simulink model "ImuCalibrator3Pass"  (R2018a)
settings: Solver=FixedStepDiscrete  StartTime=0.0  StopTime=inf  FixedStep=1/Fss  RelTol=1e-3
PreLoadFcn:
  | busDef
  | Fss = 1125;
  | Fss = 2100;
InitFcn:
  | modelDef = getModelDef(true);
undefined symbols (not defined in the file or in its folder): df, dw, Ggyr, Macc, Mgyr, numStates
libraries: simulink x15, vrlib x15, dspsigops x6, dspindex x6, dspinverses x6, dspstat3 x3, simulink_extras x3, dspmtrx3 x3, dspsrcs4 x3, dspmathops x3, dspswit3 x1
(part 3 of 4)

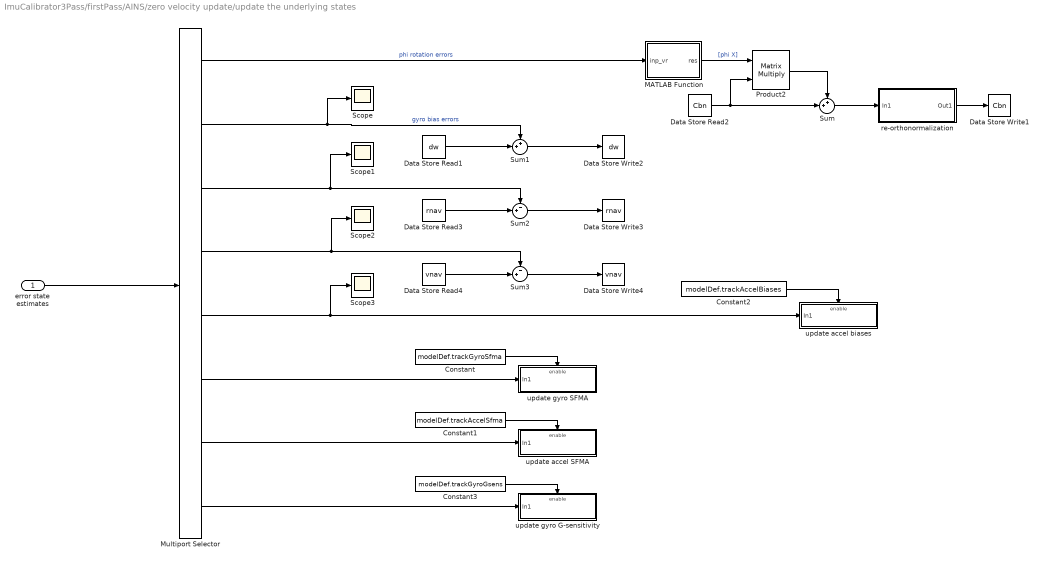
== system ImuCalibrator3Pass/firstPass/AINS/zero velocity update/update the underlying states ==
  " error state estimates" : Inport
  Constant : Constant  Value=modelDef.trackGyroSfma
  Constant1 : Constant  Value=modelDef.trackAccelSfma
  Constant2 : Constant  Value=modelDef.trackAccelBiases
  Constant3 : Constant  Value=modelDef.trackGyroGsens
  Data Store Read1 : DataStoreRead  DataStoreName=dw
  Data Store Read2 : DataStoreRead  DataStoreName=Cbn
  Data Store Read3 : DataStoreRead  DataStoreName=rnav
  Data Store Read4 : DataStoreRead  DataStoreName=vnav
  Data Store Write1 : DataStoreWrite  DataStoreName=Cbn
  Data Store Write2 : DataStoreWrite  DataStoreName=dw
  Data Store Write3 : DataStoreWrite  DataStoreName=rnav
  Data Store Write4 : DataStoreWrite  DataStoreName=vnav
  MATLAB Function : MATLAB Function  TreatAsAtomicUnit=on
  Multiport Selector : dspindex/Multiport Selector  rowsOrCols=Rows  idxCellArray={ 1:3, 4:6, 7:9, 10:12, 13:15, 16:24, 25:33, 34:42 }  idxErrMode=Clip Index
  Product2 : Product  Multiplication=Matrix(*)
  Scope{,1..3} (4 alike) : Scope
  Sum : Sum  Inputs=++|
  Sum1 : Sum  Inputs=++|
  Sum2 : Sum  Inputs=-+|
  Sum3 : Sum  Inputs=-+|
  re-orthonormalization : Subsystem  TreatAsAtomicUnit=on
  update accel SFMA : Subsystem
  update accel biases : Subsystem
  update gyro G-sensitivity : Subsystem
  update gyro SFMA : Subsystem
  wires:
  Multiport Selector/4 -> Sum3/1, Scope2/1
  Multiport Selector/3 -> Sum2/1, Scope1/1
  Sum3/1 -> Data Store Write4/1
  Data Store Read4/1 -> Sum3/2
  Data Store Read3/1 -> Sum2/2
  Sum2/1 -> Data Store Write3/1
  " error state estimates"/1 -> Multiport Selector/1
  Multiport Selector/2 -> Sum1/1, Scope/1  "gyro bias errors"
  Sum1/1 -> Data Store Write2/1
  Data Store Read1/1 -> Sum1/2
  Multiport Selector/1 -> MATLAB Function/1(inp_vr)  "phi rotation errors"
  re-orthonormalization/1(Out1) -> Data Store Write1/1
  Data Store Read2/1 -> Sum/2, Product2/2
  Sum/1 -> re-orthonormalization/1(In1)
  Product2/1 -> Sum/1
  MATLAB Function/1(res) -> Product2/1  "[phi X]"
  Constant/1 -> update gyro SFMA/Enable
  Multiport Selector/6 -> update gyro SFMA/1(In1)
  Constant1/1 -> update accel SFMA/Enable
  Multiport Selector/7 -> update accel SFMA/1(In1)
  Multiport Selector/5 -> update accel biases/1(In1), Scope3/1
  Constant2/1 -> update accel biases/Enable
  Constant3/1 -> update gyro G-sensitivity/Enable
  Multiport Selector/8 -> update gyro G-sensitivity/1(In1)

== system ImuCalibrator3Pass/secondPass/AINS/compass meas update/update the Cbn with the errors ==
  phi  rotation errors : Inport
  Data Store Read2 : DataStoreRead  DataStoreName=Cbn
  Data Store Write1 : DataStoreWrite  DataStoreName=Cbn
  MATLAB Function : MATLAB Function  TreatAsAtomicUnit=on
  Product2 : Product  Multiplication=Matrix(*)
  Sum : Sum  Inputs=++|
  re-orthonormalization : Subsystem  TreatAsAtomicUnit=on
  wires:
  MATLAB Function/1(res) -> Product2/1  "[phi X]"
  Product2/1 -> Sum/1
  Sum/1 -> re-orthonormalization/1(In1)
  phi  rotation errors/1 -> MATLAB Function/1(inp_vr)
  Data Store Read2/1 -> Product2/2, Sum/2
  re-orthonormalization/1(Out1) -> Data Store Write1/1

== system ImuCalibrator3Pass/secondPass/AINS/gravity meas update/update the Cbn and b_g with the errors ==
  " error state estimates" : Inport
  Data Store Read1 : DataStoreRead  DataStoreName=dw
  Data Store Read2 : DataStoreRead  DataStoreName=Cbn
  Data Store Read3 : DataStoreRead  DataStoreName=rnav
  Data Store Read4 : DataStoreRead  DataStoreName=vnav
  Data Store Read5 : DataStoreRead  DataStoreName=df
  Data Store Read6 : DataStoreRead  DataStoreName=Macc
  Data Store Read7 : DataStoreRead  DataStoreName=Mgyr
  Data Store Write1 : DataStoreWrite  DataStoreName=Cbn
  Data Store Write2 : DataStoreWrite  DataStoreName=dw
  Data Store Write3 : DataStoreWrite  DataStoreName=rnav
  Data Store Write4 : DataStoreWrite  DataStoreName=vnav
  Data Store Write5 : DataStoreWrite  DataStoreName=df
  Data Store Write6 : DataStoreWrite  DataStoreName=Macc
  Data Store Write7 : DataStoreWrite  DataStoreName=Mgyr
  MATLAB Function : MATLAB Function  TreatAsAtomicUnit=on
  Multiport Selector : dspindex/Multiport Selector  rowsOrCols=Rows  idxCellArray={ 1:3, 4:6, 7:9, 10:12, 13:15, 16:24, 25:33 }  idxErrMode=Clip Index
  Product2 : Product  Multiplication=Matrix(*)
  Reshape : Reshape  OutputDimensionality=Customize  OutputDimensions=[3,3]
  Reshape1 : Reshape  OutputDimensionality=Customize  OutputDimensions=[3,3]
  Sum{,1..6} (7 alike) : Sum  Inputs=++|
  re-orthonormalization : Subsystem  TreatAsAtomicUnit=on
  wires:
  Reshape1/1 -> Sum6/1
  Multiport Selector/7 -> Reshape1/1
  Reshape/1 -> Sum5/1
  Multiport Selector/6 -> Reshape/1
  Data Store Read7/1 -> Sum6/2
  Sum6/1 -> Data Store Write7/1
  Sum5/1 -> Data Store Write6/1
  Data Store Read6/1 -> Sum5/2
  Multiport Selector/5 -> Sum4/1
  Data Store Read5/1 -> Sum4/2
  Sum4/1 -> Data Store Write5/1
  Multiport Selector/4 -> Sum3/1
  Multiport Selector/3 -> Sum2/1
  Sum3/1 -> Data Store Write4/1
  Data Store Read4/1 -> Sum3/2
  Data Store Read3/1 -> Sum2/2
  Sum2/1 -> Data Store Write3/1
  " error state estimates"/1 -> Multiport Selector/1
  Multiport Selector/2 -> Sum1/1  "gyro bias errors"
  Sum1/1 -> Data Store Write2/1
  Data Store Read1/1 -> Sum1/2
  Multiport Selector/1 -> MATLAB Function/1(inp_vr)  "phi rotation errors"
  re-orthonormalization/1(Out1) -> Data Store Write1/1
  Data Store Read2/1 -> Sum/2, Product2/2
  Sum/1 -> re-orthonormalization/1(In1)
  Product2/1 -> Sum/1
  MATLAB Function/1(res) -> Product2/1  "[phi X]"

== system ImuCalibrator3Pass/secondPass/AINS/initialize states and covariances/INITIALIZED = 1 ==
  Enable : EnablePort  ShowOutputPort=on
  Constant : Constant
  Data Store Write : DataStoreWrite  DataStoreName=INITIALIZED
  Out1 : Outport  OutputWhenDisabled=reset  InitialOutput=false
  wires:
  Enable/1 -> Out1/1
  Constant/1 -> Data Store Write/1

== system ImuCalibrator3Pass/secondPass/AINS/initialize states and covariances/calc Cbn ==
  f^b : Inport
  Enable : EnablePort  ShowOutputPort=on
  Constant : Constant  Value=[1 0 0]
  Cross Product : vrlib/Utilities/Cross Product
      settings: SourceProductBaseCode=VR
  Cross Product1 : vrlib/Utilities/Cross Product
      settings: SourceProductBaseCode=VR
  Gain : Gain  Gain=-1
  Matrix Concatenate : Concatenate  NumInputs=3  Mode=Multidimensional array
  Normalize Vector : vrlib/Utilities/Normalize Vector  maxzero=0
      settings: SourceProductName=Simulink 3D Animation  SourceProductBaseCode=VR
  Normalize Vector1 : vrlib/Utilities/Normalize Vector  maxzero=0
      settings: SourceProductName=Simulink 3D Animation  SourceProductBaseCode=VR
  Normalize Vector2 : vrlib/Utilities/Normalize Vector  maxzero=0
      settings: SourceProductName=Simulink 3D Animation  SourceProductBaseCode=VR
  Out1 : Outport  OutputWhenDisabled=reset  InitialOutput=false
  Cbn : Outport  Port=2
  wires:
  Enable/1 -> Out1/1
  Matrix Concatenate/1 -> Cbn/1
  Normalize Vector2/1 -> Matrix Concatenate/3
  Normalize Vector1/1 -> Matrix Concatenate/2
  Normalize Vector/1 -> Matrix Concatenate/1
  Cross Product1/1 -> Normalize Vector/1  "north^b"
  Cross Product/1 -> Cross Product1/1, Normalize Vector1/1  "east^b"
  Constant/1 -> Cross Product/2
  Gain/1 -> Cross Product/1, Cross Product1/2, Normalize Vector2/1  "down^b"
  f^b/1 -> Gain/1  "up"

== system ImuCalibrator3Pass/secondPass/AINS/initialize states and covariances/set P ==
  Enable : EnablePort  ShowOutputPort=on
  Data Store Write : DataStoreWrite  DataStoreName=P
  Gain : Gain
  Gain2 : Gain
  Gain3 : Gain
  MATLAB Function1 : MATLAB Function  TreatAsAtomicUnit=on
  "initial position error, m rms" : Constant  Value=[0.01; 0.01; 0.01]  VectorParams1D=off
  "initial rotation error, rad rms" : Constant  Value=[0.1; 0.1; 0.1]  VectorParams1D=off
  "initial vel error, m/s" : Constant  Value=[0.01; 0.01; 0.01]  VectorParams1D=off
  Out1 : Outport  OutputWhenDisabled=reset  InitialOutput=false
  wires:
  Enable/1 -> Out1/1
  Gain3/1 -> MATLAB Function1/3(initialVelUncert)
  "initial vel error, m/s"/1 -> Gain3/1
  Gain2/1 -> MATLAB Function1/2(initialPosUncert)
  Gain/1 -> MATLAB Function1/1(initialRotUncert)
  "initial position error, m rms"/1 -> Gain2/1
  "initial rotation error, rad rms"/1 -> Gain/1
  MATLAB Function1/1(P0) -> Data Store Write/1

== system ImuCalibrator3Pass/secondPass/AINS/initialize states and covariances/set states ==
  Cbn : Inport
  Enable : EnablePort  ShowOutputPort=on
  Constant{,1..3} (4 alike) : Constant  Value=[0;0;0]
  Constant4 : Constant  Value=[0 0 0; 0 0 0; 0 0 0]  VectorParams1D=off
  Constant5 : Constant  Value=[0 0 0; 0 0 0; 0 0 0]  VectorParams1D=off
  Constant6 : Constant  Value=[1 0 0; 0 1 0; 0 0 1]  VectorParams1D=off
  Constant7 : Constant  Value=[1 0 0; 0 1 0; 0 0 1]  VectorParams1D=off
  Constant8 : Constant  Value=[0 0 0; 0 0 0; 0 0 0]  VectorParams1D=off
  Data Store Write : DataStoreWrite  DataStoreName=dw
  Data Store Write1 : DataStoreWrite  DataStoreName=df
  Data Store Write2 : DataStoreWrite  DataStoreName=vnav
  Data Store Write3 : DataStoreWrite  DataStoreName=rnav
  Data Store Write4 : DataStoreWrite  DataStoreName=Macc
  Data Store Write5 : DataStoreWrite  DataStoreName=Mgyr
  Data Store Write6 : DataStoreWrite  DataStoreName=IplusMinv_acc
  Data Store Write7 : DataStoreWrite  DataStoreName=IplusMinv_gyr
  Data Store Write8 : DataStoreWrite  DataStoreName=Cbn
  Data Store Write9 : DataStoreWrite  DataStoreName=Ggyr
  Out1 : Outport  OutputWhenDisabled=reset  InitialOutput=false
  wires:
  Constant8/1 -> Data Store Write9/1
  Cbn/1 -> Data Store Write8/1
  Enable/1 -> Out1/1
  Constant7/1 -> Data Store Write7/1
  Constant6/1 -> Data Store Write6/1
  Constant5/1 -> Data Store Write5/1
  Constant4/1 -> Data Store Write4/1
  Constant3/1 -> Data Store Write3/1
  Constant2/1 -> Data Store Write2/1
  Constant1/1 -> Data Store Write1/1
  Constant/1 -> Data Store Write/1

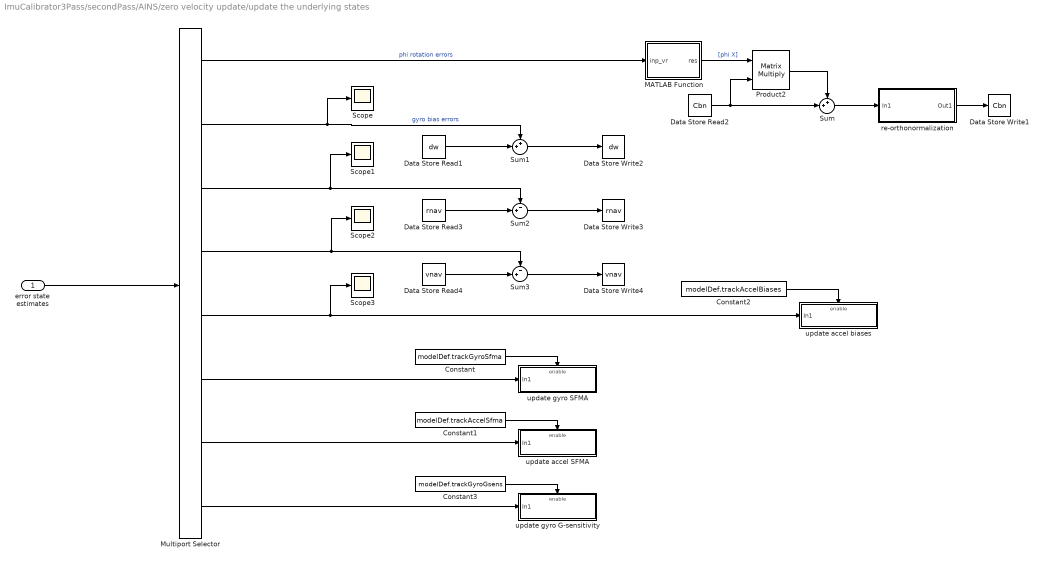
== system ImuCalibrator3Pass/secondPass/AINS/zero velocity update/update the underlying states ==
  " error state estimates" : Inport
  Constant : Constant  Value=modelDef.trackGyroSfma
  Constant1 : Constant  Value=modelDef.trackAccelSfma
  Constant2 : Constant  Value=modelDef.trackAccelBiases
  Constant3 : Constant  Value=modelDef.trackGyroGsens
  Data Store Read1 : DataStoreRead  DataStoreName=dw
  Data Store Read2 : DataStoreRead  DataStoreName=Cbn
  Data Store Read3 : DataStoreRead  DataStoreName=rnav
  Data Store Read4 : DataStoreRead  DataStoreName=vnav
  Data Store Write1 : DataStoreWrite  DataStoreName=Cbn
  Data Store Write2 : DataStoreWrite  DataStoreName=dw
  Data Store Write3 : DataStoreWrite  DataStoreName=rnav
  Data Store Write4 : DataStoreWrite  DataStoreName=vnav
  MATLAB Function : MATLAB Function  TreatAsAtomicUnit=on
  Multiport Selector : dspindex/Multiport Selector  rowsOrCols=Rows  idxCellArray={ 1:3, 4:6, 7:9, 10:12, 13:15, 16:24, 25:33, 34:42 }  idxErrMode=Clip Index
  Product2 : Product  Multiplication=Matrix(*)
  Scope{,1..3} (4 alike) : Scope
  Sum : Sum  Inputs=++|
  Sum1 : Sum  Inputs=++|
  Sum2 : Sum  Inputs=-+|
  Sum3 : Sum  Inputs=-+|
  re-orthonormalization : Subsystem  TreatAsAtomicUnit=on
  update accel SFMA : Subsystem
  update accel biases : Subsystem
  update gyro G-sensitivity : Subsystem
  update gyro SFMA : Subsystem
  wires:
  Multiport Selector/8 -> update gyro G-sensitivity/1(In1)
  Constant3/1 -> update gyro G-sensitivity/Enable
  Constant2/1 -> update accel biases/Enable
  Multiport Selector/5 -> Scope3/1, update accel biases/1(In1)
  Multiport Selector/7 -> update accel SFMA/1(In1)
  Constant1/1 -> update accel SFMA/Enable
  Multiport Selector/6 -> update gyro SFMA/1(In1)
  Constant/1 -> update gyro SFMA/Enable
  MATLAB Function/1(res) -> Product2/1  "[phi X]"
  Product2/1 -> Sum/1
  Sum/1 -> re-orthonormalization/1(In1)
  Data Store Read2/1 -> Product2/2, Sum/2
  re-orthonormalization/1(Out1) -> Data Store Write1/1
  Multiport Selector/1 -> MATLAB Function/1(inp_vr)  "phi rotation errors"
  Data Store Read1/1 -> Sum1/2
  Sum1/1 -> Data Store Write2/1
  Multiport Selector/2 -> Scope/1, Sum1/1  "gyro bias errors"
  " error state estimates"/1 -> Multiport Selector/1
  Sum2/1 -> Data Store Write3/1
  Data Store Read3/1 -> Sum2/2
  Data Store Read4/1 -> Sum3/2
  Sum3/1 -> Data Store Write4/1
  Multiport Selector/3 -> Scope1/1, Sum2/1
  Multiport Selector/4 -> Scope2/1, Sum3/1

== system ImuCalibrator3Pass/thirdPass/AINS/compass meas update/update the Cbn with the errors ==
  phi  rotation errors : Inport
  Data Store Read2 : DataStoreRead  DataStoreName=Cbn
  Data Store Write1 : DataStoreWrite  DataStoreName=Cbn
  MATLAB Function : MATLAB Function  TreatAsAtomicUnit=on
  Product2 : Product  Multiplication=Matrix(*)
  Sum : Sum  Inputs=++|
  re-orthonormalization : Subsystem  TreatAsAtomicUnit=on
  wires:
  re-orthonormalization/1(Out1) -> Data Store Write1/1
  Data Store Read2/1 -> Sum/2, Product2/2
  phi  rotation errors/1 -> MATLAB Function/1(inp_vr)
  Sum/1 -> re-orthonormalization/1(In1)
  Product2/1 -> Sum/1
  MATLAB Function/1(res) -> Product2/1  "[phi X]"

== system ImuCalibrator3Pass/thirdPass/AINS/gravity meas update/update the Cbn and b_g with the errors ==
  " error state estimates" : Inport
  Data Store Read1 : DataStoreRead  DataStoreName=dw
  Data Store Read2 : DataStoreRead  DataStoreName=Cbn
  Data Store Read3 : DataStoreRead  DataStoreName=rnav
  Data Store Read4 : DataStoreRead  DataStoreName=vnav
  Data Store Read5 : DataStoreRead  DataStoreName=df
  Data Store Read6 : DataStoreRead  DataStoreName=Macc
  Data Store Read7 : DataStoreRead  DataStoreName=Mgyr
  Data Store Write1 : DataStoreWrite  DataStoreName=Cbn
  Data Store Write2 : DataStoreWrite  DataStoreName=dw
  Data Store Write3 : DataStoreWrite  DataStoreName=rnav
  Data Store Write4 : DataStoreWrite  DataStoreName=vnav
  Data Store Write5 : DataStoreWrite  DataStoreName=df
  Data Store Write6 : DataStoreWrite  DataStoreName=Macc
  Data Store Write7 : DataStoreWrite  DataStoreName=Mgyr
  MATLAB Function : MATLAB Function  TreatAsAtomicUnit=on
  Multiport Selector : dspindex/Multiport Selector  rowsOrCols=Rows  idxCellArray={ 1:3, 4:6, 7:9, 10:12, 13:15, 16:24, 25:33 }  idxErrMode=Clip Index
  Product2 : Product  Multiplication=Matrix(*)
  Reshape : Reshape  OutputDimensionality=Customize  OutputDimensions=[3,3]
  Reshape1 : Reshape  OutputDimensionality=Customize  OutputDimensions=[3,3]
  Sum{,1..6} (7 alike) : Sum  Inputs=++|
  re-orthonormalization : Subsystem  TreatAsAtomicUnit=on
  wires:
  MATLAB Function/1(res) -> Product2/1  "[phi X]"
  Product2/1 -> Sum/1
  Sum/1 -> re-orthonormalization/1(In1)
  Data Store Read2/1 -> Product2/2, Sum/2
  re-orthonormalization/1(Out1) -> Data Store Write1/1
  Multiport Selector/1 -> MATLAB Function/1(inp_vr)  "phi rotation errors"
  Data Store Read1/1 -> Sum1/2
  Sum1/1 -> Data Store Write2/1
  Multiport Selector/2 -> Sum1/1  "gyro bias errors"
  " error state estimates"/1 -> Multiport Selector/1
  Sum2/1 -> Data Store Write3/1
  Data Store Read3/1 -> Sum2/2
  Data Store Read4/1 -> Sum3/2
  Sum3/1 -> Data Store Write4/1
  Multiport Selector/3 -> Sum2/1
  Multiport Selector/4 -> Sum3/1
  Sum4/1 -> Data Store Write5/1
  Data Store Read5/1 -> Sum4/2
  Multiport Selector/5 -> Sum4/1
  Data Store Read6/1 -> Sum5/2
  Sum5/1 -> Data Store Write6/1
  Sum6/1 -> Data Store Write7/1
  Data Store Read7/1 -> Sum6/2
  Multiport Selector/6 -> Reshape/1
  Reshape/1 -> Sum5/1
  Multiport Selector/7 -> Reshape1/1
  Reshape1/1 -> Sum6/1

== system ImuCalibrator3Pass/thirdPass/AINS/initialize states and covariances/INITIALIZED = 1 ==
  Enable : EnablePort  ShowOutputPort=on
  Constant : Constant
  Data Store Write : DataStoreWrite  DataStoreName=INITIALIZED
  Out1 : Outport  OutputWhenDisabled=reset  InitialOutput=false
  wires:
  Constant/1 -> Data Store Write/1
  Enable/1 -> Out1/1

== system ImuCalibrator3Pass/thirdPass/AINS/initialize states and covariances/calc Cbn ==
  f^b : Inport
  Enable : EnablePort  ShowOutputPort=on
  Constant : Constant  Value=[1 0 0]
  Cross Product : vrlib/Utilities/Cross Product
      settings: SourceProductBaseCode=VR
  Cross Product1 : vrlib/Utilities/Cross Product
      settings: SourceProductBaseCode=VR
  Gain : Gain  Gain=-1
  Matrix Concatenate : Concatenate  NumInputs=3  Mode=Multidimensional array
  Normalize Vector : vrlib/Utilities/Normalize Vector  maxzero=0
      settings: SourceProductName=Simulink 3D Animation  SourceProductBaseCode=VR
  Normalize Vector1 : vrlib/Utilities/Normalize Vector  maxzero=0
      settings: SourceProductName=Simulink 3D Animation  SourceProductBaseCode=VR
  Normalize Vector2 : vrlib/Utilities/Normalize Vector  maxzero=0
      settings: SourceProductName=Simulink 3D Animation  SourceProductBaseCode=VR
  Out1 : Outport  OutputWhenDisabled=reset  InitialOutput=false
  Cbn : Outport  Port=2
  wires:
  f^b/1 -> Gain/1  "up"
  Gain/1 -> Normalize Vector2/1, Cross Product1/2, Cross Product/1  "down^b"
  Constant/1 -> Cross Product/2
  Cross Product/1 -> Normalize Vector1/1, Cross Product1/1  "east^b"
  Cross Product1/1 -> Normalize Vector/1  "north^b"
  Normalize Vector/1 -> Matrix Concatenate/1
  Normalize Vector1/1 -> Matrix Concatenate/2
  Normalize Vector2/1 -> Matrix Concatenate/3
  Matrix Concatenate/1 -> Cbn/1
  Enable/1 -> Out1/1

== system ImuCalibrator3Pass/thirdPass/AINS/initialize states and covariances/set P ==
  Enable : EnablePort  ShowOutputPort=on
  Data Store Write : DataStoreWrite  DataStoreName=P
  Gain : Gain
  Gain2 : Gain
  Gain3 : Gain
  MATLAB Function1 : MATLAB Function  TreatAsAtomicUnit=on
  "initial position error, m rms" : Constant  Value=[0.01; 0.01; 0.01]  VectorParams1D=off
  "initial rotation error, rad rms" : Constant  Value=[0.1; 0.1; 0.1]  VectorParams1D=off
  "initial vel error, m/s" : Constant  Value=[0.01; 0.01; 0.01]  VectorParams1D=off
  Out1 : Outport  OutputWhenDisabled=reset  InitialOutput=false
  wires:
  MATLAB Function1/1(P0) -> Data Store Write/1
  "initial rotation error, rad rms"/1 -> Gain/1
  "initial position error, m rms"/1 -> Gain2/1
  Gain/1 -> MATLAB Function1/1(initialRotUncert)
  Gain2/1 -> MATLAB Function1/2(initialPosUncert)
  "initial vel error, m/s"/1 -> Gain3/1
  Gain3/1 -> MATLAB Function1/3(initialVelUncert)
  Enable/1 -> Out1/1

== system ImuCalibrator3Pass/thirdPass/AINS/initialize states and covariances/set states ==
  Cbn : Inport
  Enable : EnablePort  ShowOutputPort=on
  Constant{,1..3} (4 alike) : Constant  Value=[0;0;0]
  Constant4 : Constant  Value=[0 0 0; 0 0 0; 0 0 0]  VectorParams1D=off
  Constant5 : Constant  Value=[0 0 0; 0 0 0; 0 0 0]  VectorParams1D=off
  Constant6 : Constant  Value=[1 0 0; 0 1 0; 0 0 1]  VectorParams1D=off
  Constant7 : Constant  Value=[1 0 0; 0 1 0; 0 0 1]  VectorParams1D=off
  Constant8 : Constant  Value=[0 0 0; 0 0 0; 0 0 0]  VectorParams1D=off
  Data Store Write : DataStoreWrite  DataStoreName=dw
  Data Store Write1 : DataStoreWrite  DataStoreName=df
  Data Store Write2 : DataStoreWrite  DataStoreName=vnav
  Data Store Write3 : DataStoreWrite  DataStoreName=rnav
  Data Store Write4 : DataStoreWrite  DataStoreName=Macc
  Data Store Write5 : DataStoreWrite  DataStoreName=Mgyr
  Data Store Write6 : DataStoreWrite  DataStoreName=IplusMinv_acc
  Data Store Write7 : DataStoreWrite  DataStoreName=IplusMinv_gyr
  Data Store Write8 : DataStoreWrite  DataStoreName=Cbn
  Data Store Write9 : DataStoreWrite  DataStoreName=Ggyr
  Out1 : Outport  OutputWhenDisabled=reset  InitialOutput=false
  wires:
  Constant/1 -> Data Store Write/1
  Constant1/1 -> Data Store Write1/1
  Constant2/1 -> Data Store Write2/1
  Constant3/1 -> Data Store Write3/1
  Constant4/1 -> Data Store Write4/1
  Constant5/1 -> Data Store Write5/1
  Constant6/1 -> Data Store Write6/1
  Constant7/1 -> Data Store Write7/1
  Enable/1 -> Out1/1
  Cbn/1 -> Data Store Write8/1
  Constant8/1 -> Data Store Write9/1

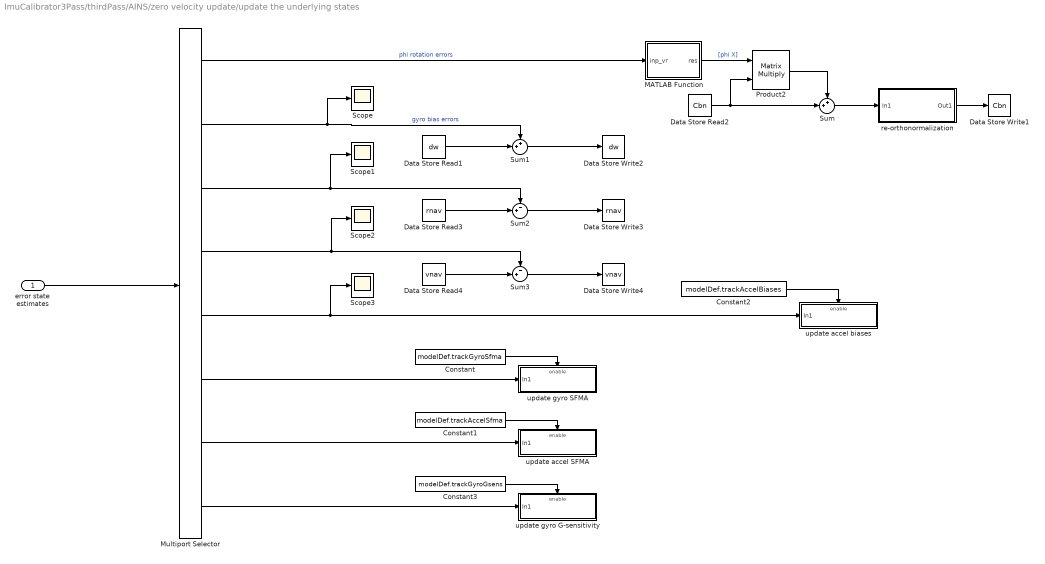
== system ImuCalibrator3Pass/thirdPass/AINS/zero velocity update/update the underlying states ==
  " error state estimates" : Inport
  Constant : Constant  Value=modelDef.trackGyroSfma
  Constant1 : Constant  Value=modelDef.trackAccelSfma
  Constant2 : Constant  Value=modelDef.trackAccelBiases
  Constant3 : Constant  Value=modelDef.trackGyroGsens
  Data Store Read1 : DataStoreRead  DataStoreName=dw
  Data Store Read2 : DataStoreRead  DataStoreName=Cbn
  Data Store Read3 : DataStoreRead  DataStoreName=rnav
  Data Store Read4 : DataStoreRead  DataStoreName=vnav
  Data Store Write1 : DataStoreWrite  DataStoreName=Cbn
  Data Store Write2 : DataStoreWrite  DataStoreName=dw
  Data Store Write3 : DataStoreWrite  DataStoreName=rnav
  Data Store Write4 : DataStoreWrite  DataStoreName=vnav
  MATLAB Function : MATLAB Function  TreatAsAtomicUnit=on
  Multiport Selector : dspindex/Multiport Selector  rowsOrCols=Rows  idxCellArray={ 1:3, 4:6, 7:9, 10:12, 13:15, 16:24, 25:33, 34:42 }  idxErrMode=Clip Index
  Product2 : Product  Multiplication=Matrix(*)
  Scope{,1..3} (4 alike) : Scope
  Sum : Sum  Inputs=++|
  Sum1 : Sum  Inputs=++|
  Sum2 : Sum  Inputs=-+|
  Sum3 : Sum  Inputs=-+|
  re-orthonormalization : Subsystem  TreatAsAtomicUnit=on
  update accel SFMA : Subsystem
  update accel biases : Subsystem
  update gyro G-sensitivity : Subsystem
  update gyro SFMA : Subsystem
  wires:
  Multiport Selector/4 -> Sum3/1, Scope2/1
  Multiport Selector/3 -> Sum2/1, Scope1/1
  Sum3/1 -> Data Store Write4/1
  Data Store Read4/1 -> Sum3/2
  Data Store Read3/1 -> Sum2/2
  Sum2/1 -> Data Store Write3/1
  " error state estimates"/1 -> Multiport Selector/1
  Multiport Selector/2 -> Sum1/1, Scope/1  "gyro bias errors"
  Sum1/1 -> Data Store Write2/1
  Data Store Read1/1 -> Sum1/2
  Multiport Selector/1 -> MATLAB Function/1(inp_vr)  "phi rotation errors"
  re-orthonormalization/1(Out1) -> Data Store Write1/1
  Data Store Read2/1 -> Sum/2, Product2/2
  Sum/1 -> re-orthonormalization/1(In1)
  Product2/1 -> Sum/1
  MATLAB Function/1(res) -> Product2/1  "[phi X]"
  Constant/1 -> update gyro SFMA/Enable
  Multiport Selector/6 -> update gyro SFMA/1(In1)
  Constant1/1 -> update accel SFMA/Enable
  Multiport Selector/7 -> update accel SFMA/1(In1)
  Multiport Selector/5 -> update accel biases/1(In1), Scope3/1
  Constant2/1 -> update accel biases/Enable
  Constant3/1 -> update gyro G-sensitivity/Enable
  Multiport Selector/8 -> update gyro G-sensitivity/1(In1)

== system ImuCalibrator3Pass/firstPass/AINS/compass meas update/update the Cbn with the errors/re-orthonormalization ==
  note: Cfixed = C + 0.5(I-CC')C
  note: from http://www.dtic.mil/dtic/tr/fulltext/u2/p003621.pdf page 12
  In1 : Inport
  C*C' : Product  Multiplication=Matrix(*)
  C*C'1 : Product  Multiplication=Matrix(*)
  Constant : Constant  Value=eye(3)
  Display : Display
  Gain : Gain  Gain=1/2
  Permute Dimensions : PermuteDimensions
  Sum : Sum  Inputs=|++
  Sum1 : Sum  Inputs=|+-
  Out1 : Outport
  wires:
  C*C'1/1 -> Gain/1
  Sum1/1 -> C*C'1/1
  Gain/1 -> Sum/2
  Constant/1 -> Sum1/1
  C*C'/1 -> Sum1/2
  Permute Dimensions/1 -> C*C'/2
  Sum/1 -> Out1/1, Display/1
  In1/1 -> Sum/1, C*C'1/2, C*C'/1, Permute Dimensions/1

== system ImuCalibrator3Pass/firstPass/AINS/gravity meas update/update the Cbn and b_g with the errors/re-orthonormalization ==
  note: from http://www.dtic.mil/dtic/tr/fulltext/u2/p003621.pdf page 12
  note: Cfixed = C + 0.5(I-CC')C
  In1 : Inport
  C*C' : Product  Multiplication=Matrix(*)
  C*C'1 : Product  Multiplication=Matrix(*)
  Constant : Constant  Value=eye(3)
  Gain : Gain  Gain=1/2
  Permute Dimensions : PermuteDimensions
  Sum : Sum  Inputs=|++
  Sum1 : Sum  Inputs=|+-
  Out1 : Outport
  wires:
  In1/1 -> Permute Dimensions/1, C*C'/1, C*C'1/2, Sum/1
  Sum/1 -> Out1/1
  Permute Dimensions/1 -> C*C'/2
  C*C'/1 -> Sum1/2
  Constant/1 -> Sum1/1
  Gain/1 -> Sum/2
  Sum1/1 -> C*C'1/1
  C*C'1/1 -> Gain/1

== system ImuCalibrator3Pass/firstPass/AINS/zero velocity update/update the underlying states/re-orthonormalization ==
  note: Cfixed = C + 0.5(I-CC')C
  note: from http://www.dtic.mil/dtic/tr/fulltext/u2/p003621.pdf page 12
  In1 : Inport
  C*C' : Product  Multiplication=Matrix(*)
  C*C'1 : Product  Multiplication=Matrix(*)
  Constant : Constant  Value=eye(3)
  Gain : Gain  Gain=1/2
  Permute Dimensions : PermuteDimensions
  Sum : Sum  Inputs=|++
  Sum1 : Sum  Inputs=|+-
  Out1 : Outport
  wires:
  C*C'1/1 -> Gain/1
  Sum1/1 -> C*C'1/1
  Gain/1 -> Sum/2
  Constant/1 -> Sum1/1
  C*C'/1 -> Sum1/2
  Permute Dimensions/1 -> C*C'/2
  Sum/1 -> Out1/1
  In1/1 -> Sum/1, C*C'1/2, C*C'/1, Permute Dimensions/1

== system ImuCalibrator3Pass/firstPass/AINS/zero velocity update/update the underlying states/update accel SFMA ==
  In1 : Inport
  Enable : EnablePort
  " LU Inverse" : dspinverses/ LU Inverse
      settings: SourceProductName=DSP System Toolbox
  Bias : Bias  Bias=eye(3)
  Data Store Read6 : DataStoreRead  DataStoreName=Macc
  Data Store Write6 : DataStoreWrite  DataStoreName=Macc
  Data Store Write9 : DataStoreWrite  DataStoreName=IplusMinv_acc
  Reshape : Reshape  OutputDimensionality=Customize  OutputDimensions=[3,3]
  Sum5 : Sum  Inputs=++|
  wires:
  Sum5/1 -> Bias/1, Data Store Write6/1
  Data Store Read6/1 -> Sum5/2
  Reshape/1 -> Sum5/1
  In1/1 -> Reshape/1
  Bias/1 -> " LU Inverse"/1
  " LU Inverse"/1 -> Data Store Write9/1

== system ImuCalibrator3Pass/firstPass/AINS/zero velocity update/update the underlying states/update accel biases ==
  In1 : Inport
  Enable : EnablePort
  Data Store Read5 : DataStoreRead  DataStoreName=df
  Data Store Write5 : DataStoreWrite  DataStoreName=df
  Sum4 : Sum  Inputs=++|
  wires:
  Sum4/1 -> Data Store Write5/1
  Data Store Read5/1 -> Sum4/2
  In1/1 -> Sum4/1

== system ImuCalibrator3Pass/firstPass/AINS/zero velocity update/update the underlying states/update gyro G-sensitivity ==
  In1 : Inport
  Enable : EnablePort
  Data Store Read7 : DataStoreRead  DataStoreName=Ggyr
  Data Store Write7 : DataStoreWrite  DataStoreName=Ggyr
  Reshape1 : Reshape  OutputDimensionality=Customize  OutputDimensions=[3,3]
  Sum6 : Sum  Inputs=++|
  wires:
  Sum6/1 -> Data Store Write7/1
  In1/1 -> Reshape1/1
  Reshape1/1 -> Sum6/1
  Data Store Read7/1 -> Sum6/2

== system ImuCalibrator3Pass/firstPass/AINS/zero velocity update/update the underlying states/update gyro SFMA ==
  In1 : Inport
  Enable : EnablePort
  " LU Inverse1" : dspinverses/ LU Inverse
      settings: SourceProductName=DSP System Toolbox
  Bias1 : Bias  Bias=eye(3)
  Data Store Read7 : DataStoreRead  DataStoreName=Mgyr
  Data Store Write7 : DataStoreWrite  DataStoreName=Mgyr
  Data Store Write8 : DataStoreWrite  DataStoreName=IplusMinv_gyr
  Reshape1 : Reshape  OutputDimensionality=Customize  OutputDimensions=[3,3]
  Sum6 : Sum  Inputs=++|
  wires:
  Sum6/1 -> Bias1/1, Data Store Write7/1
  In1/1 -> Reshape1/1
  Reshape1/1 -> Sum6/1
  Data Store Read7/1 -> Sum6/2
  Bias1/1 -> " LU Inverse1"/1
  " LU Inverse1"/1 -> Data Store Write8/1

== system ImuCalibrator3Pass/secondPass/AINS/compass meas update/update the Cbn with the errors/re-orthonormalization ==
  note: from http://www.dtic.mil/dtic/tr/fulltext/u2/p003621.pdf page 12
  note: Cfixed = C + 0.5(I-CC')C
  In1 : Inport
  C*C' : Product  Multiplication=Matrix(*)
  C*C'1 : Product  Multiplication=Matrix(*)
  Constant : Constant  Value=eye(3)
  Display : Display
  Gain : Gain  Gain=1/2
  Permute Dimensions : PermuteDimensions
  Sum : Sum  Inputs=|++
  Sum1 : Sum  Inputs=|+-
  Out1 : Outport
  wires:
  In1/1 -> Permute Dimensions/1, C*C'/1, C*C'1/2, Sum/1
  Sum/1 -> Display/1, Out1/1
  Permute Dimensions/1 -> C*C'/2
  C*C'/1 -> Sum1/2
  Constant/1 -> Sum1/1
  Gain/1 -> Sum/2
  Sum1/1 -> C*C'1/1
  C*C'1/1 -> Gain/1

== system ImuCalibrator3Pass/secondPass/AINS/gravity meas update/update the Cbn and b_g with the errors/re-orthonormalization ==
  note: Cfixed = C + 0.5(I-CC')C
  note: from http://www.dtic.mil/dtic/tr/fulltext/u2/p003621.pdf page 12
  In1 : Inport
  C*C' : Product  Multiplication=Matrix(*)
  C*C'1 : Product  Multiplication=Matrix(*)
  Constant : Constant  Value=eye(3)
  Gain : Gain  Gain=1/2
  Permute Dimensions : PermuteDimensions
  Sum : Sum  Inputs=|++
  Sum1 : Sum  Inputs=|+-
  Out1 : Outport
  wires:
  C*C'1/1 -> Gain/1
  Sum1/1 -> C*C'1/1
  Gain/1 -> Sum/2
  Constant/1 -> Sum1/1
  C*C'/1 -> Sum1/2
  Permute Dimensions/1 -> C*C'/2
  Sum/1 -> Out1/1
  In1/1 -> Sum/1, C*C'1/2, C*C'/1, Permute Dimensions/1

== system ImuCalibrator3Pass/secondPass/AINS/zero velocity update/update the underlying states/re-orthonormalization ==
  note: from http://www.dtic.mil/dtic/tr/fulltext/u2/p003621.pdf page 12
  note: Cfixed = C + 0.5(I-CC')C
  In1 : Inport
  C*C' : Product  Multiplication=Matrix(*)
  C*C'1 : Product  Multiplication=Matrix(*)
  Constant : Constant  Value=eye(3)
  Gain : Gain  Gain=1/2
  Permute Dimensions : PermuteDimensions
  Sum : Sum  Inputs=|++
  Sum1 : Sum  Inputs=|+-
  Out1 : Outport
  wires:
  In1/1 -> Permute Dimensions/1, C*C'/1, C*C'1/2, Sum/1
  Sum/1 -> Out1/1
  Permute Dimensions/1 -> C*C'/2
  C*C'/1 -> Sum1/2
  Constant/1 -> Sum1/1
  Gain/1 -> Sum/2
  Sum1/1 -> C*C'1/1
  C*C'1/1 -> Gain/1

== system ImuCalibrator3Pass/secondPass/AINS/zero velocity update/update the underlying states/update accel SFMA ==
  In1 : Inport
  Enable : EnablePort
  " LU Inverse" : dspinverses/ LU Inverse
      settings: SourceProductName=DSP System Toolbox
  Bias : Bias  Bias=eye(3)
  Data Store Read6 : DataStoreRead  DataStoreName=Macc
  Data Store Write6 : DataStoreWrite  DataStoreName=Macc
  Data Store Write9 : DataStoreWrite  DataStoreName=IplusMinv_acc
  Reshape : Reshape  OutputDimensionality=Customize  OutputDimensions=[3,3]
  Sum5 : Sum  Inputs=++|
  wires:
  " LU Inverse"/1 -> Data Store Write9/1
  Bias/1 -> " LU Inverse"/1
  In1/1 -> Reshape/1
  Reshape/1 -> Sum5/1
  Data Store Read6/1 -> Sum5/2
  Sum5/1 -> Data Store Write6/1, Bias/1

== system ImuCalibrator3Pass/secondPass/AINS/zero velocity update/update the underlying states/update accel biases ==
  In1 : Inport
  Enable : EnablePort
  Data Store Read5 : DataStoreRead  DataStoreName=df
  Data Store Write5 : DataStoreWrite  DataStoreName=df
  Sum4 : Sum  Inputs=++|
  wires:
  In1/1 -> Sum4/1
  Data Store Read5/1 -> Sum4/2
  Sum4/1 -> Data Store Write5/1

== system ImuCalibrator3Pass/secondPass/AINS/zero velocity update/update the underlying states/update gyro G-sensitivity ==
  In1 : Inport
  Enable : EnablePort
  Data Store Read7 : DataStoreRead  DataStoreName=Ggyr
  Data Store Write7 : DataStoreWrite  DataStoreName=Ggyr
  Reshape1 : Reshape  OutputDimensionality=Customize  OutputDimensions=[3,3]
  Sum6 : Sum  Inputs=++|
  wires:
  Data Store Read7/1 -> Sum6/2
  Reshape1/1 -> Sum6/1
  In1/1 -> Reshape1/1
  Sum6/1 -> Data Store Write7/1

== system ImuCalibrator3Pass/secondPass/AINS/zero velocity update/update the underlying states/update gyro SFMA ==
  In1 : Inport
  Enable : EnablePort
  " LU Inverse1" : dspinverses/ LU Inverse
      settings: SourceProductName=DSP System Toolbox
  Bias1 : Bias  Bias=eye(3)
  Data Store Read7 : DataStoreRead  DataStoreName=Mgyr
  Data Store Write7 : DataStoreWrite  DataStoreName=Mgyr
  Data Store Write8 : DataStoreWrite  DataStoreName=IplusMinv_gyr
  Reshape1 : Reshape  OutputDimensionality=Customize  OutputDimensions=[3,3]
  Sum6 : Sum  Inputs=++|
  wires:
  " LU Inverse1"/1 -> Data Store Write8/1
  Bias1/1 -> " LU Inverse1"/1
  Data Store Read7/1 -> Sum6/2
  Reshape1/1 -> Sum6/1
  In1/1 -> Reshape1/1
  Sum6/1 -> Data Store Write7/1, Bias1/1

== system ImuCalibrator3Pass/thirdPass/AINS/compass meas update/update the Cbn with the errors/re-orthonormalization ==
  note: Cfixed = C + 0.5(I-CC')C
  note: from http://www.dtic.mil/dtic/tr/fulltext/u2/p003621.pdf page 12
  In1 : Inport
  C*C' : Product  Multiplication=Matrix(*)
  C*C'1 : Product  Multiplication=Matrix(*)
  Constant : Constant  Value=eye(3)
  Display : Display
  Gain : Gain  Gain=1/2
  Permute Dimensions : PermuteDimensions
  Sum : Sum  Inputs=|++
  Sum1 : Sum  Inputs=|+-
  Out1 : Outport
  wires:
  C*C'1/1 -> Gain/1
  Sum1/1 -> C*C'1/1
  Gain/1 -> Sum/2
  Constant/1 -> Sum1/1
  C*C'/1 -> Sum1/2
  Permute Dimensions/1 -> C*C'/2
  Sum/1 -> Out1/1, Display/1
  In1/1 -> Sum/1, C*C'1/2, C*C'/1, Permute Dimensions/1

== system ImuCalibrator3Pass/thirdPass/AINS/gravity meas update/update the Cbn and b_g with the errors/re-orthonormalization ==
  note: from http://www.dtic.mil/dtic/tr/fulltext/u2/p003621.pdf page 12
  note: Cfixed = C + 0.5(I-CC')C
  In1 : Inport
  C*C' : Product  Multiplication=Matrix(*)
  C*C'1 : Product  Multiplication=Matrix(*)
  Constant : Constant  Value=eye(3)
  Gain : Gain  Gain=1/2
  Permute Dimensions : PermuteDimensions
  Sum : Sum  Inputs=|++
  Sum1 : Sum  Inputs=|+-
  Out1 : Outport
  wires:
  In1/1 -> Permute Dimensions/1, C*C'/1, C*C'1/2, Sum/1
  Sum/1 -> Out1/1
  Permute Dimensions/1 -> C*C'/2
  C*C'/1 -> Sum1/2
  Constant/1 -> Sum1/1
  Gain/1 -> Sum/2
  Sum1/1 -> C*C'1/1
  C*C'1/1 -> Gain/1

== system ImuCalibrator3Pass/thirdPass/AINS/zero velocity update/update the underlying states/re-orthonormalization ==
  note: Cfixed = C + 0.5(I-CC')C
  note: from http://www.dtic.mil/dtic/tr/fulltext/u2/p003621.pdf page 12
  In1 : Inport
  C*C' : Product  Multiplication=Matrix(*)
  C*C'1 : Product  Multiplication=Matrix(*)
  Constant : Constant  Value=eye(3)
  Gain : Gain  Gain=1/2
  Permute Dimensions : PermuteDimensions
  Sum : Sum  Inputs=|++
  Sum1 : Sum  Inputs=|+-
  Out1 : Outport
  wires:
  C*C'1/1 -> Gain/1
  Sum1/1 -> C*C'1/1
  Gain/1 -> Sum/2
  Constant/1 -> Sum1/1
  C*C'/1 -> Sum1/2
  Permute Dimensions/1 -> C*C'/2
  Sum/1 -> Out1/1
  In1/1 -> Sum/1, C*C'1/2, C*C'/1, Permute Dimensions/1

== system ImuCalibrator3Pass/thirdPass/AINS/zero velocity update/update the underlying states/update accel SFMA ==
  In1 : Inport
  Enable : EnablePort
  " LU Inverse" : dspinverses/ LU Inverse
      settings: SourceProductName=DSP System Toolbox
  Bias : Bias  Bias=eye(3)
  Data Store Read6 : DataStoreRead  DataStoreName=Macc
  Data Store Write6 : DataStoreWrite  DataStoreName=Macc
  Data Store Write9 : DataStoreWrite  DataStoreName=IplusMinv_acc
  Reshape : Reshape  OutputDimensionality=Customize  OutputDimensions=[3,3]
  Sum5 : Sum  Inputs=++|
  wires:
  Sum5/1 -> Bias/1, Data Store Write6/1
  Data Store Read6/1 -> Sum5/2
  Reshape/1 -> Sum5/1
  In1/1 -> Reshape/1
  Bias/1 -> " LU Inverse"/1
  " LU Inverse"/1 -> Data Store Write9/1

== system ImuCalibrator3Pass/thirdPass/AINS/zero velocity update/update the underlying states/update accel biases ==
  In1 : Inport
  Enable : EnablePort
  Data Store Read5 : DataStoreRead  DataStoreName=df
  Data Store Write5 : DataStoreWrite  DataStoreName=df
  Sum4 : Sum  Inputs=++|
  wires:
  Sum4/1 -> Data Store Write5/1
  Data Store Read5/1 -> Sum4/2
  In1/1 -> Sum4/1

== system ImuCalibrator3Pass/thirdPass/AINS/zero velocity update/update the underlying states/update gyro G-sensitivity ==
  In1 : Inport
  Enable : EnablePort
  Data Store Read7 : DataStoreRead  DataStoreName=Ggyr
  Data Store Write7 : DataStoreWrite  DataStoreName=Ggyr
  Reshape1 : Reshape  OutputDimensionality=Customize  OutputDimensions=[3,3]
  Sum6 : Sum  Inputs=++|
  wires:
  Sum6/1 -> Data Store Write7/1
  In1/1 -> Reshape1/1
  Reshape1/1 -> Sum6/1
  Data Store Read7/1 -> Sum6/2

== system ImuCalibrator3Pass/thirdPass/AINS/zero velocity update/update the underlying states/update gyro SFMA ==
  In1 : Inport
  Enable : EnablePort
  " LU Inverse1" : dspinverses/ LU Inverse
      settings: SourceProductName=DSP System Toolbox
  Bias1 : Bias  Bias=eye(3)
  Data Store Read7 : DataStoreRead  DataStoreName=Mgyr
  Data Store Write7 : DataStoreWrite  DataStoreName=Mgyr
  Data Store Write8 : DataStoreWrite  DataStoreName=IplusMinv_gyr
  Reshape1 : Reshape  OutputDimensionality=Customize  OutputDimensions=[3,3]
  Sum6 : Sum  Inputs=++|
  wires:
  Sum6/1 -> Bias1/1, Data Store Write7/1
  In1/1 -> Reshape1/1
  Reshape1/1 -> Sum6/1
  Data Store Read7/1 -> Sum6/2
  Bias1/1 -> " LU Inverse1"/1
  " LU Inverse1"/1 -> Data Store Write8/1

== matlab function ImuCalibrator3Pass/firstPass/AINS/INS/MATLAB Function2 ==
  data: Cbn input; Cbn_new output; w input; dt input
function Cbn_new = update_dcm(Cbn, w, dt)

% Update attitude according to TW p.312 approximated to sixth order

rot=w*dt;
rot_norm=norm(rot);
sr_a=1-(rot_norm^2/6)+(rot_norm^4/120);
sr_b=(1/2)-(rot_norm^2/24)+(rot_norm^4/720);
mx_a=eye(3)+sr_a*skew(rot)+sr_b*skew(rot)*skew(rot);

Cbn_new=Cbn*mx_a;


function res=skew(inp_vr)
res=[0 			-inp_vr(3)	inp_vr(2); ...
     inp_vr(3)	0			-inp_vr(1);...
	 -inp_vr(2)	inp_vr(1)	0];

== matlab function ImuCalibrator3Pass/firstPass/AINS/report output/MATLAB Function3 ==
  data: Cbn input; eul output size=[3,1]
function eul = dcm2euler(Cbn)

%DCM is Cbn (transforms vectors from b to n)
%eul defined as zyx sequence (yaw,pitch,roll),  but listed in
%roll,pitch,yaw order


pitch=asin(-Cbn(3,1));  %pitch is assumed to be [-pi pi]. singular at pi. use ad-hoc methods to remedy this deficiency
roll=atan2(Cbn(3,2), Cbn(3,3));
heading = atan2(Cbn(2,1), Cbn(1,1));
eul=[roll;pitch;heading];

== matlab function ImuCalibrator3Pass/firstPass/AINS/gravity meas update/update the Cbn and b_g with the errors/MATLAB Function ==
  data: inp_vr input; res output
function res=skew(inp_vr)
res=[0 			-inp_vr(3)	inp_vr(2); ...
     inp_vr(3)	0			-inp_vr(1);...
	 -inp_vr(2)	inp_vr(1)	0];

== matlab function ImuCalibrator3Pass/firstPass/AINS/gravity meas update/MATLAB Function1 ==
  data: S output; P input; K output; H input; R input
function [S,K] = calcKalmanGain(P, H, R)

PHT = P*H';
S = H*PHT + R;
K = PHT/S;

== matlab function ImuCalibrator3Pass/firstPass/AINS/MATLAB Function ==
  data: w input; stilltime output; f input; Dt input; favgs output; wavgs output
function [stilltime, favgs, wavgs] = update_stilltime(w, f, Dt)

persistent stillt wavg favg stillcycles wsigmas fsigmas;

if isempty(wavg)
    stillt = 0;
    stillcycles = 0;
    wavg = w;
    favg = f;
    wsigmas = 0.02*[1;1;1];%%0.01*[1;1;1];
    fsigmas = 0.4*[1;1;1];%0.2*[1;1;1];
end

if all(abs(f-favg) < 3*fsigmas) && all(abs(w-wavg) < 3*wsigmas)  % increment the stilltimes
    stillt = stillt + Dt;
    stillcycles = stillcycles + 1;
%     % simple recursive mean (weighting all the samples equally):
%     wavg = ((stillcycles-1)*wavg + w)/stillcycles;
%     favg = ((stillcycles-1)*favg + f)/stillcycles;

%     % recursive mean with each sample weighted by the stillcycles when it came in:
%     wavg = ((stillcycles-1)*wavg + 2*w)/(stillcycles+1);
%     favg = ((stillcycles-1)*favg + 2*f)/(stillcycles+1);

    % start with stilltime weighting and switch back to simple recursive mean after 1 second to reduce noise:
    if stillt < 1
        wavg = ((stillcycles-1)*wavg + 2*w)/(stillcycles+1);
        favg = ((stillcycles-1)*favg + 2*f)/(stillcycles+1);
    else
        wavg = ((stillcycles-1)*wavg + w)/stillcycles;
        favg = ((stillcycles-1)*favg + f)/stillcycles;
    end        
else  %reset stilltime
    stillt = 0;
    stillcycles = 0;
    wavg = w;
    favg = f;
end    

stilltime = stillt;
favgs = favg;
wavgs = wavg;

== matlab function ImuCalibrator3Pass/firstPass/AINS/time update/MATLAB Function ==
  data: omega input; Q output size=[modelDef.numStates, modelDef.numStates]; f_ib input; Dt input; Cbn input; modelDef parameter; imuPar parameter
function Q  = calculate_Q(omega, f_ib, Dt, Cbn, modelDef, imuPar)

% order of the states:
% 1:3   phi
% 4:6   dw
% 7:9   dr
% 10:12 dv
% 13:15 df  (if modelDef.trackAccelBiases)
% 16:24 dM_gyro in column-major order (if modelDef.trackGyroSfma)
% 25:33 dM_accel in column-major order (if modelDef.trackAccelSfma)

Q = zeros(modelDef.numStates, modelDef.numStates);

omega = reshape(omega,3,1); 
f_ib = reshape(f_ib, 3,1);

Qphi = diag((imuPar.gyroArwRadPerRtSec^2)*[Dt Dt Dt]);  
Qdw = diag((imuPar.gyroBrwRadPerSecPerRtSec^2)*[Dt Dt Dt]);
Qdv = diag((imuPar.accelVrwMetersPerSecPerRtSec^2)*[Dt Dt Dt]);
Qdf = diag((imuPar.accelBrwMetersPerSec2PerRtSec^2)*[Dt Dt Dt]);


%bump up Q for unmodelled states
if ~modelDef.trackGyroSfma % gyro scale factor and misalignment not tracked
   gyroSfSigmaBod = imuPar.gyroScaleUncert*omega;
   gyroMaSigmaBod = imuPar.gyroAlignUncert*sqrt(omega'*omega*[1 1 1]-omega'.*omega');   
   QgyroMa = Cbn*diag(gyroMaSigmaBod.^2)*Cbn'*Dt; 
   QgyroSf = Cbn*diag(gyroSfSigmaBod.^2)*Cbn'*Dt; 
   Qphi = Qphi + QgyroMa + QgyroSf;   
end

if ~modelDef.trackGyroGsens %  gyro g sensitivity not tracked 
   gGsensSigmaBod = imuPar.gyroGsensUncert*sqrt(f_ib'*f_ib*[1 1 1]-f_ib'.*f_ib');   
   QgGsens = Cbn*diag(gGsensSigmaBod.^2)*Cbn'*Dt; 
   Qphi = Qphi + QgGsens;   
end

if ~modelDef.trackAccelSfma  % accel scale factor and misalignment not tracked
   accelSfSigmaBod = imuPar.accelScaleUncert*f_ib;
   accelMaSigmaBod = imuPar.accelAlignUncert*sqrt(f_ib'*f_ib*[1 1 1]-f_ib'.*f_ib');   
   QaccelMa = Cbn*diag(accelMaSigmaBod.^2)*Cbn'*Dt; 
   QaccelSf = Cbn*diag(accelSfSigmaBod.^2)*Cbn'*Dt; 
   Qdv = Qdv + QaccelMa + QaccelSf;   
end

Q(1:3, 1:3) = Qphi;
Q(4:6, 4:6) = Qdw;
Q(10:12, 10:12) = Qdv;
Q(13:15, 13:15) = Qdf;

== matlab function ImuCalibrator3Pass/firstPass/AINS/time update/MATLAB Function1 ==
  data: imuPar output Bus: imuPar
function imuPar = imuPar

imuPar.gyroArwDegPerRtHr = 0.25;
imuPar.gyroArwRadPerRtSec = imuPar.gyroArwDegPerRtHr * pi/180/60;
imuPar.gyroBrwDegPerHrPerRtHr = 0;
imuPar.gyroBrwRadPerSecPerRtSec = imuPar.gyroBrwDegPerHrPerRtHr * pi/180/3600/60;
imuPar.gyroScaleUncertainty = 0.001;
imuPar.gyroAlignUncertainty = 0.01;
imuPar.gyroGsensUncertainty = 0.001;

== matlab function ImuCalibrator3Pass/firstPass/AINS/time update/MATLAB Function2 ==
  settings: updateMethod=DISCRETE  sampleTime=inf
  data: modelDef output Bus: modelDef; numStates input
function modelDef = modelDef(numStates)

modelDef.trackAccelBiases = true;
modelDef.trackAccelSfma = true;
modelDef.trackGyroSfma = true;
modelDef.trackGyroGsens = false;

modelDef.numStates = numStates;

== matlab function ImuCalibrator3Pass/firstPass/AINS/time update/MATLAB Function3 ==
  data: omega input; Phi output size=[modelDef.numStates, modelDef.numStates]; fbod input; Dt input; Cbn input; modelDef parameter
function Phi  = calculate_Phi(omega, fbod, Dt, Cbn, modelDef)

% order of the states:
% 1:3   phi
% 4:6   dw
% 7:9   dr
% 10:12 dv
% 13:15 df  (if modelDef.trackAccelBiases)
% 16:24 dM_gyro in column-major order (if modelDef.trackGyroSfma)
% 25:33 dM_accel in column-major order (if modelDef.trackAccelSfma)
% 34:42 dG_gyro in column-major order (if modelDef.trackGyroGsens)

Phi = eye(modelDef.numStates);

DtC = Dt*Cbn;

Phi(1:3,4:6) = -DtC;  % propagate dw to phi
Phi(7:9, 10:12) = Dt*eye(3);  % propagate dv to dr
Phi(10:12, 1:3) = Dt*skew(Cbn*fbod);  % propagate phi to dv

if modelDef.trackAccelBiases
    Phi(10:12, 13:15) = DtC;   % propagate df to dv
end

if modelDef.trackGyroSfma  % propagate dM_gyro to phi
    Phi(1:3, 16:18) = -DtC*omega(1);
    Phi(1:3, 19:21) = -DtC*omega(2);
    Phi(1:3, 22:24) = -DtC*omega(3);
end

if modelDef.trackAccelSfma  % propagate dM_accel to dv
    Phi(10:12, 25:27) = DtC*fbod(1);
    Phi(10:12, 28:30) = DtC*fbod(2);
    Phi(10:12, 31:33) = DtC*fbod(3);
end

if modelDef.trackGyroGsens  % propagate dG_gyro to phi
    Phi(1:3, 34:36) = -DtC*fbod(1);
    Phi(1:3, 37:39) = -DtC*fbod(2);
    Phi(1:3, 40:42) = -DtC*fbod(3);
end

function res=skew(inp_vr)
res=[0 			-inp_vr(3)	inp_vr(2); ...
     inp_vr(3)	0			-inp_vr(1);...
	 -inp_vr(2)	inp_vr(1)	0];

== matlab function ImuCalibrator3Pass/firstPass/AINS/zero velocity update/MATLAB Function1 ==
  data: S output; P input; K output; H input; R input
function [S,K] = calcKalmanGain(P, H, R)

PHT = P*H';
S = H*PHT + R;
K = PHT/S;

== matlab function ImuCalibrator3Pass/firstPass/printTime/MATLAB Function ==
  data: u input
function  printTime(u)
%#codegen

% using fileId = 1  only generates a printf in the generated code
% fileId = 2 also causes prints in the matlab console

fprintf(2, "\r 1st pass: %f sec", u);

== matlab function ImuCalibrator3Pass/firstPass/AINS/initialize states and covariances/set P/MATLAB Function1 ==
  data: initialRotUncert input; initialPosUncert input; initialVelUncert input; P0 output size=[modelDef.numStates, modelDef.numStates]; modelDef parameter; imuPar parameter
function P0  = calculate_P0(initialRotUncert, initialPosUncert, initialVelUncert, modelDef, imuPar)

% order of the states:
% 1:3   phi
% 4:6   dw
% 7:9   dr
% 10:12 dv
% 13:15 df  (if modelDef.trackAccelBiases)
% 16:24 dM_gyro in column-major order (if modelDef.trackGyroSfma)
% 25:33 dM_accel in column-major order (if modelDef.trackAccelSfma)
% 34:42 dG_gyro in column-major order (if modelDef.trackGyroGsens)

P0 = zeros(modelDef.numStates, modelDef.numStates);

P0(1:3, 1:3) = diag(initialRotUncert.^2);
P0(4:6, 4:6) = eye(3)*(imuPar.gyroBiasUncert.^2);
P0(7:9, 7:9) = diag(initialPosUncert.^2);
P0(10:12, 10:12) = diag(initialVelUncert.^2);


if modelDef.trackAccelBiases
    P0(13:15, 13:15) = eye(3)*(imuPar.accelBiasUncert.^2);
end

if modelDef.trackGyroSfma  
    vec9 = ones(9,1)*imuPar.gyroAlignUncert^2;
    vec9([1 5 9]) = imuPar.gyroScaleUncert^2;
    P0(16:24, 16:24) = diag(vec9);
end

if modelDef.trackAccelSfma  % propagate dM_accel to dv
    vec9 = ones(9,1)*imuPar.accelAlignUncert^2;
    vec9([1 5 9]) = imuPar.accelScaleUncert^2;
    if modelDef.accelDefinesExtrinsics
        vec9([4 7]) = 0.0001^2; % x accel has no misalignment so picks up no component of y or z accelerations
        vec9(8) = 0.0001^2;  % y accel has no tilt out of xy plane, so picks up no component of z acceleration
    end
    P0(25:33, 25:33) = diag(vec9);
end

if modelDef.trackGyroGsens
    vec9 = ones(9,1)*imuPar.gyroGsensUncert^2;
    P0(34:42, 34:42) = diag(vec9);
end

== matlab function ImuCalibrator3Pass/firstPass/AINS/gravity meas update/MATLAB Function3 ==
  data: P input; Pplus output; K input; H input; R input; IminKH output
function [Pplus, IminKH] = josephCovarianceUpdate(P, K, H, R)

IminKH = eye(size(P)) - K*H;
Pplus = IminKH*P*IminKH' + K*R*K';

== matlab function ImuCalibrator3Pass/firstPass/AINS/zero velocity update/MATLAB Function3 ==
  data: P input; Pplus output; K input; H input; R input; IminKH output
function [Pplus, IminKH] = josephCovarianceUpdate(P, K, H, R)

IminKH = eye(size(P)) - K*H;
Pplus = IminKH*P*IminKH' + K*R*K';

== matlab function ImuCalibrator3Pass/firstPass/AINS/zero velocity update/update the underlying states/MATLAB Function ==
  data: inp_vr input; res output
function res=skew(inp_vr)
res=[0 			-inp_vr(3)	inp_vr(2); ...
     inp_vr(3)	0			-inp_vr(1);...
	 -inp_vr(2)	inp_vr(1)	0];

== matlab function ImuCalibrator3Pass/firstPass/AINS/report output/MATLAB Function1 ==
  data: Cbn input; quat output size=[4,1]
function quat=dcm2quat(Cbn)

%dcm (Cba) to quaternion (qba)
%Cba:B to A transformation matrix
%qba:B to A quaternion

%Implementation of savage(3-47)


tr=Cbn(1,1)+Cbn(2,2)+Cbn(3,3);
Pa=1+tr;
Pb=1+2*Cbn(1,1)-tr;
Pc=1+2*Cbn(2,2)-tr;
Pd=1+2*Cbn(3,3)-tr;

quat=zeros(4,1);
if (Pa>=Pb && Pa>=Pc && Pa>=Pd)
    quat(1)=0.5*sqrt(Pa);
    quat(2)=(Cbn(3,2)-Cbn(2,3))/4/quat(1);
    quat(3)=(Cbn(1,3)-Cbn(3,1))/4/quat(1);
    quat(4)=(Cbn(2,1)-Cbn(1,2))/4/quat(1);
elseif (Pb>=Pc && Pb>=Pd)
    quat(2)=0.5*sqrt(Pb);
    quat(3)=(Cbn(2,1)+Cbn(1,2))/4/quat(2);
    quat(4)=(Cbn(1,3)+Cbn(3,1))/4/quat(2);
    quat(1)=(Cbn(3,2)-Cbn(2,3))/4/quat(2);
elseif (Pc>=Pd)
    quat(3)=0.5*sqrt(Pc);
    quat(4)=(Cbn(3,2)+Cbn(2,3))/4/quat(3);
    quat(1)=(Cbn(1,3)-Cbn(3,1))/4/quat(3);
    quat(2)=(Cbn(2,1)+Cbn(1,2))/4/quat(3);
else
    quat(4)=0.5*sqrt(Pd);
    quat(1)=(Cbn(2,1)-Cbn(1,2))/4/quat(4);
    quat(2)=(Cbn(1,3)+Cbn(3,1))/4/quat(4);
    quat(3)=(Cbn(3,2)+Cbn(2,3))/4/quat(4);
end

if (quat(1)<=0)
    quat=-quat;
end
